simulink model "RealLifeTrainModel"  (R2024a)
settings: Solver=ode1  StartTime=0.0  StopTime=Inf  FixedStep=0.001  RelTol=1e-3
PostLoadFcn:
  | , if any(exist('dsrtsu_mdlpostloadfcn', 'file') ~= 0), dsrtsu_mdlpostloadfcn('Execute', bdroot); end,
InitFcn:
  | , if any(exist('rtifpga_mdlclblib', 'file') ~= 0), rtifpga_mdlclblib('Init', bdroot); end,
undefined symbols (not defined in the file): DiscIntNeverNeededParam
libraries: deeplib x29, svdutilitieslib x28, simulink x8, eeGeneralControl x8, rti1202lib_adc_class1 x6, rti1202serlib x5, spsEdgeDetectorLib x5, rtiemclib x2, rti1202lib_dac_class1 x1
(part 3 of 8)

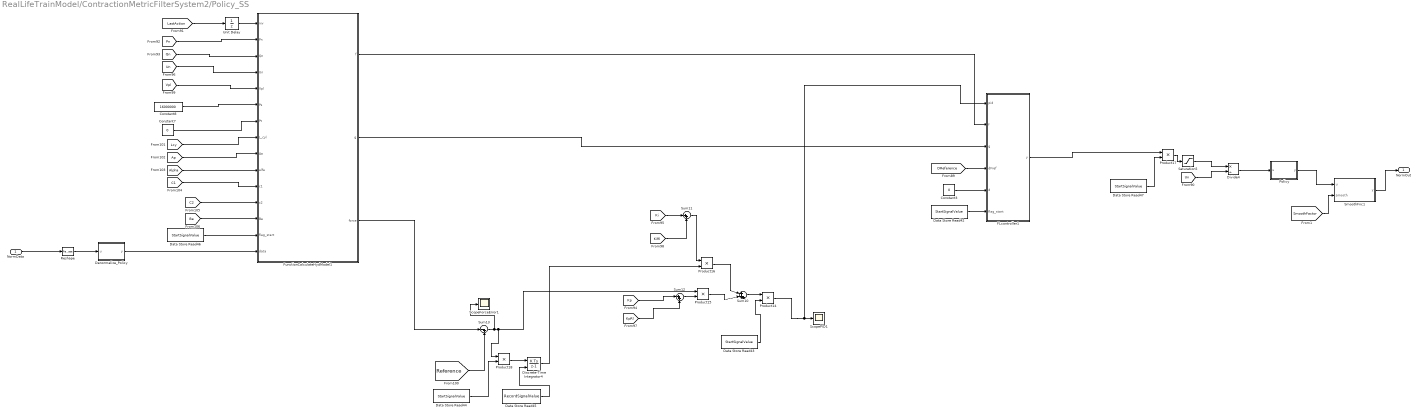
== system RealLifeTrainModel/ContractionMetricFilterSystem2/Policy_SS ==
  NormData : Inport
  Constant3 : Constant  Value=0
  Constant7 : Constant  Value=0
  Constant8 : Constant  Value=16000000
  Data Store Read{42..44,46..47} (5 alike) : DataStoreRead  DataStoreName=StartSignalValue  IndexOptions=Index vector (dialog)  Indices=1  OutputSizes=1
  Data Store Read45 : DataStoreRead  DataStoreName=RecordSignalValue  IndexOptions=Index vector (dialog)  Indices=1  OutputSizes=1
  Denormalize_Policy : MATLAB Function  TreatAsAtomicUnit=on
  Discrete-Time Integrator4 : DiscreteIntegrator  ExternalReset=falling  SampleTime=-1  ICPrevOutput=DiscIntNeverNeededParam  ICPrevScaledInput=DiscIntNeverNeededParam
  Divide4 : Product  Inputs=*/
  FLcontroller1 : MATLAB Function  TreatAsAtomicUnit=on
  FunctionCalculateHydModel1 : MATLAB Function  TreatAsAtomicUnit=on
  Policy : MATLAB Function  TreatAsAtomicUnit=on
  Product{14..18} (5 alike) : Product
  Reshape : Reshape  OutputDimensionality=Row vector (2-D)  OutputDimensions=[8,1]
  Saturation5 : Saturate  UpperLimit=str2num(get_param('Teste_PID/Un','Value'))/str2num(get_param('Teste_PID/SaturationDivider','Value'))  LowerLimit=-str2num(get_param('Teste_PID/Un','Value'))/str2num(get_param('Teste_PID/SaturationDivider','Value'))
  ScopeForceError1 : Scope
  ScopePID1 : Scope
  SmoothFnc1 : MATLAB Function  TreatAsAtomicUnit=on
  Sum10 : Sum  Inputs=|+++
  Sum11 : Sum  Inputs=|++
  Sum12 : Sum  Inputs=|++
  Sum13 : Sum  Inputs=|-+
  Unit Delay : UnitDelay  SampleTime=-1  HasFrameUpgradeWarning=on
  NormOut : Outport
  wires:
  FunctionCalculateHydModel1/3(force) -> Sum13/1
  [Vpl] -> FunctionCalculateHydModel1/5(Vpl)
  Data Store Read45/1 -> Discrete-Time Integrator4/2
  Sum13/1 -> ScopeForceError1/1, Product15/1, Product18/1
  [Alpha] -> FunctionCalculateHydModel1/10(alfa)
  [C2] -> FunctionCalculateHydModel1/12(c2)
  Data Store Read42/1 -> FLcontroller1/6(flag_start)
  [Be] -> FunctionCalculateHydModel1/13(Be)
  [Lcy] -> FunctionCalculateHydModel1/8(L_cyl)
  Data Store Read43/1 -> Product14/2
  [Ap] -> FunctionCalculateHydModel1/9(Aa)
  Product15/1 -> Sum10/2
  Data Store Read44/1 -> Product18/2
  Product18/1 -> Discrete-Time Integrator4/1
  [KpRl] -> Sum12/2
  [Reference] -> Sum13/2
  Constant8/1 -> FunctionCalculateHydModel1/6(Ps)
  Product14/1 -> FLcontroller1/1(pid), ScopePID1/1
  Sum11/1 -> Product16/1
  Sum12/1 -> Product15/2
  Saturation5/1 -> Divide4/1
  [Un] -> Divide4/2
  FLcontroller1/1(y) -> Product17/1
  Denormalize_Policy/1(y) -> FunctionCalculateHydModel1/15(data)
  Sum10/1 -> Product14/1
  [C1] -> FunctionCalculateHydModel1/11(c1)
  Discrete-Time Integrator4/1 -> Product16/2
  [Pn] -> FunctionCalculateHydModel1/2(Pn)
  [LastAction] -> Unit Delay/1
  [Kp] -> Sum12/1
  [Ki] -> Sum11/1
  Constant7/1 -> FunctionCalculateHydModel1/7(Pt)
  Divide4/1 -> Policy/1(u)
  [Qn] -> FunctionCalculateHydModel1/3(Qn)
  Constant3/1 -> FLcontroller1/5(d)
  [KiRl] -> Sum11/2
  Data Store Read47/1 -> Product17/2
  Product16/1 -> Sum10/1
  FunctionCalculateHydModel1/2(g) -> FLcontroller1/3(g)
  Product17/1 -> Saturation5/1
  [DReference] -> FLcontroller1/4(dFref)
  FunctionCalculateHydModel1/1(f) -> FLcontroller1/2(f)
  [Un] -> FunctionCalculateHydModel1/4(Un)
  Data Store Read46/1 -> FunctionCalculateHydModel1/14(flag_start)
  NormData/1 -> Reshape/1
  Reshape/1 -> Denormalize_Policy/1(u)
  Unit Delay/1 -> FunctionCalculateHydModel1/1(ixv)
  [SmoothFactor] -> SmoothFnc1/2(smooth)
  Policy/1(y) -> SmoothFnc1/1(u)
  SmoothFnc1/1(y) -> NormOut/1

== system RealLifeTrainModel/ContractionMetricFilterSystem3/CalcK ==
  State : Inport
  Constant : Constant
  Constant1 : Constant  Value=2
  Constant2 : Constant  Value=3
  Constant3 : Constant  Value=4
  Constant4 : Constant  Value=5
  Constant5 : Constant  Value=6
  Constant6 : Constant  Value=7
  Constant7 : Constant  Value=8
  IndidualGrad1 : Subsystem
  IndidualGrad10 : Subsystem
  IndidualGrad2 : Subsystem
  IndidualGrad3 : Subsystem
  IndidualGrad4 : Subsystem
  IndidualGrad5 : Subsystem
  IndidualGrad6 : Subsystem
  IndidualGrad7 : Subsystem
  Mux : Mux  Inputs=8
  Policy_SS1 : Subsystem
  Reshape8 : Reshape  OutputDimensionality=Customize  OutputDimensions=[1,8]
  K : Outport
  wires:
  State/1 -> Policy_SS1/1(NormData), IndidualGrad7/1(State), IndidualGrad6/1(State), IndidualGrad5/1(State), IndidualGrad4/1(State), IndidualGrad3/1(State), IndidualGrad2/1(State), IndidualGrad1/1(State), IndidualGrad10/1(State)
  Constant/1 -> IndidualGrad10/2(Position)
  Mux/1 -> Reshape8/1
  Constant1/1 -> IndidualGrad1/2(Position)
  Constant2/1 -> IndidualGrad2/2(Position)
  Constant3/1 -> IndidualGrad3/2(Position)
  Constant4/1 -> IndidualGrad4/2(Position)
  Constant5/1 -> IndidualGrad5/2(Position)
  Constant6/1 -> IndidualGrad6/2(Position)
  Constant7/1 -> IndidualGrad7/2(Position)
  Policy_SS1/1(NormOut) -> IndidualGrad6/3(StartValue), IndidualGrad7/3(StartValue), IndidualGrad5/3(StartValue), IndidualGrad4/3(StartValue), IndidualGrad3/3(StartValue), IndidualGrad2/3(StartValue), IndidualGrad1/3(StartValue), IndidualGrad10/3(StartValue)
  IndidualGrad10/1(Grad) -> Mux/1
  IndidualGrad1/1(Grad) -> Mux/2
  IndidualGrad2/1(Grad) -> Mux/3
  IndidualGrad3/1(Grad) -> Mux/4
  IndidualGrad4/1(Grad) -> Mux/5
  IndidualGrad5/1(Grad) -> Mux/6
  IndidualGrad6/1(Grad) -> Mux/7
  IndidualGrad7/1(Grad) -> Mux/8
  Reshape8/1 -> K/1

== system RealLifeTrainModel/ContractionMetricFilterSystem3/Calc_A_B ==
  state : Inport
  Current : Inport  Port=2
  Calc_A_Grad : Subsystem
  A : Outport
  B : Outport  Port=2
  ModelPredict : Outport  Port=3
  wires:
  state/1 -> Calc_A_Grad/1(State)
  Calc_A_Grad/1(A) -> A/1
  Calc_A_Grad/2(B) -> B/1
  Current/1 -> Calc_A_Grad/2(Curent)
  Calc_A_Grad/3(ModelPredict) -> ModelPredict/1

== system RealLifeTrainModel/ContractionMetricFilterSystem3/Mdot_subsystem ==
  StartMetric : Inport
  State : Inport  Port=2
  NextState : Inport  Port=3
  Constant : Constant
  Constant1 : Constant  Value=2
  Constant2 : Constant  Value=3
  Constant3 : Constant  Value=4
  Constant4 : Constant  Value=5
  Constant5 : Constant  Value=6
  Constant6 : Constant  Value=7
  Constant7 : Constant  Value=8
  ConvertMatrix : MATLAB Function  TreatAsAtomicUnit=on
  Demux : Demux  Outputs=8
  Discrete Derivative : simulink/Discrete/Discrete Derivative  gainval=1.0  ICPrevScaledInput=0.0  OutMin=[]  OutMax=[]  OutDataType=fixdt(1, 16)  OutScaling=2^-10  DoSatur=off
  IndidualGrad1 : Subsystem
  IndidualGrad10 : Subsystem
  IndidualGrad2 : Subsystem
  IndidualGrad3 : Subsystem
  IndidualGrad4 : Subsystem
  IndidualGrad5 : Subsystem
  IndidualGrad6 : Subsystem
  IndidualGrad7 : Subsystem
  Product{,1..7} (8 alike) : Product
  Sum : Sum  Inputs=|++++++++
  Mdot : Outport
  wires:
  Constant/1 -> IndidualGrad10/2(Position)
  StartMetric/1 -> ConvertMatrix/1(M_flat)
  State/1 -> Discrete Derivative/1, IndidualGrad7/1(State), IndidualGrad6/1(State), IndidualGrad5/1(State), IndidualGrad4/1(State), IndidualGrad3/1(State), IndidualGrad2/1(State), IndidualGrad1/1(State), IndidualGrad10/1(State)
  Constant1/1 -> IndidualGrad1/2(Position)
  Constant2/1 -> IndidualGrad2/2(Position)
  Constant3/1 -> IndidualGrad3/2(Position)
  Constant4/1 -> IndidualGrad4/2(Position)
  Constant5/1 -> IndidualGrad5/2(Position)
  Constant6/1 -> IndidualGrad6/2(Position)
  Constant7/1 -> IndidualGrad7/2(Position)
  Demux/1 -> [State1]
  Demux/8 -> [State8]
  Demux/7 -> [State7]
  Demux/6 -> [State6]
  Demux/5 -> [State5]
  Demux/4 -> [State4]
  Demux/3 -> [State3]
  Demux/2 -> [State2]
  [State1] -> Product/1
  IndidualGrad10/1(Grad) -> Product/2
  Product/1 -> Sum/1
  [State2] -> Product1/1
  IndidualGrad1/1(Grad) -> Product1/2
  Product1/1 -> Sum/2
  [State3] -> Product2/1
  IndidualGrad2/1(Grad) -> Product2/2
  Product2/1 -> Sum/3
  [State4] -> Product3/1
  IndidualGrad3/1(Grad) -> Product3/2
  Product3/1 -> Sum/4
  [State5] -> Product4/1
  IndidualGrad4/1(Grad) -> Product4/2
  Product4/1 -> Sum/5
  [State6] -> Product5/1
  IndidualGrad5/1(Grad) -> Product5/2
  Product5/1 -> Sum/6
  [State7] -> Product6/1
  [State8] -> Product7/1
  IndidualGrad6/1(Grad) -> Product6/2
  Product6/1 -> Sum/7
  IndidualGrad7/1(Grad) -> Product7/2
  Product7/1 -> Sum/8
  ConvertMatrix/1(M) -> IndidualGrad7/3(StartValue), IndidualGrad6/3(StartValue), IndidualGrad5/3(StartValue), IndidualGrad4/3(StartValue), IndidualGrad3/3(StartValue), IndidualGrad2/3(StartValue), IndidualGrad1/3(StartValue), IndidualGrad10/3(StartValue)
  Sum/1 -> Mdot/1
  NextState/1 -> Demux/1

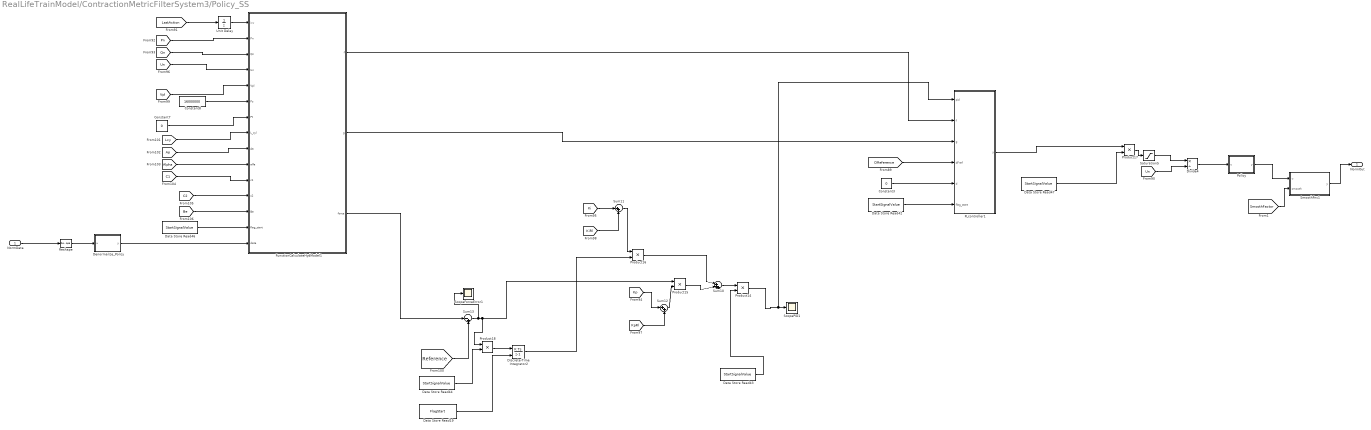
== system RealLifeTrainModel/ContractionMetricFilterSystem3/Policy_SS ==
  NormData : Inport
  Constant3 : Constant  Value=0
  Constant7 : Constant  Value=0
  Constant8 : Constant  Value=16000000
  Data Store Read19 : DataStoreRead  DataStoreName=FlagStart  IndexOptions=Index vector (dialog)  Indices=1  OutputSizes=1
  Data Store Read{42..44,46..47} (5 alike) : DataStoreRead  DataStoreName=StartSignalValue  IndexOptions=Index vector (dialog)  Indices=1  OutputSizes=1
  Denormalize_Policy : MATLAB Function  TreatAsAtomicUnit=on
  Discrete-Time Integrator2 : DiscreteIntegrator  ExternalReset=either  SampleTime=-1  ICPrevOutput=DiscIntNeverNeededParam  ICPrevScaledInput=DiscIntNeverNeededParam
  Divide4 : Product  Inputs=*/
  FLcontroller1 : MATLAB Function  TreatAsAtomicUnit=on
  FunctionCalculateHydModel1 : MATLAB Function  TreatAsAtomicUnit=on
  Policy : MATLAB Function  TreatAsAtomicUnit=on
  Product{14..18} (5 alike) : Product
  Reshape : Reshape  OutputDimensionality=Row vector (2-D)  OutputDimensions=[8,1]
  Saturation5 : Saturate  UpperLimit=str2num(get_param('Teste_PID/Un','Value'))/str2num(get_param('Teste_PID/SaturationDivider','Value'))  LowerLimit=-str2num(get_param('Teste_PID/Un','Value'))/str2num(get_param('Teste_PID/SaturationDivider','Value'))
  ScopeForceError1 : Scope
  ScopePID1 : Scope
  SmoothFnc1 : MATLAB Function  TreatAsAtomicUnit=on
  Sum10 : Sum  Inputs=|+++
  Sum11 : Sum  Inputs=|++
  Sum12 : Sum  Inputs=|++
  Sum13 : Sum  Inputs=|-+
  Unit Delay : UnitDelay  SampleTime=-1  HasFrameUpgradeWarning=on
  NormOut : Outport
  wires:
  FunctionCalculateHydModel1/3(force) -> Sum13/1
  [Vpl] -> FunctionCalculateHydModel1/5(Vpl)
  Sum13/1 -> ScopeForceError1/1, Product15/1, Product18/1
  [Alpha] -> FunctionCalculateHydModel1/10(alfa)
  [C2] -> FunctionCalculateHydModel1/12(c2)
  Data Store Read42/1 -> FLcontroller1/6(flag_start)
  [Be] -> FunctionCalculateHydModel1/13(Be)
  [Lcy] -> FunctionCalculateHydModel1/8(L_cyl)
  Data Store Read43/1 -> Product14/2
  [Ap] -> FunctionCalculateHydModel1/9(Aa)
  Product15/1 -> Sum10/2
  Data Store Read44/1 -> Product18/2
  Product18/1 -> Discrete-Time Integrator2/1
  [KpRl] -> Sum12/2
  [Reference] -> Sum13/2
  Constant8/1 -> FunctionCalculateHydModel1/6(Ps)
  Product14/1 -> FLcontroller1/1(pid), ScopePID1/1
  Sum11/1 -> Product16/1
  Sum12/1 -> Product15/2
  Saturation5/1 -> Divide4/1
  [Un] -> Divide4/2
  FLcontroller1/1(y) -> Product17/1
  Denormalize_Policy/1(y) -> FunctionCalculateHydModel1/15(data)
  Sum10/1 -> Product14/1
  [C1] -> FunctionCalculateHydModel1/11(c1)
  Discrete-Time Integrator2/1 -> Product16/2
  [Pn] -> FunctionCalculateHydModel1/2(Pn)
  [LastAction] -> Unit Delay/1
  [Kp] -> Sum12/1
  [Ki] -> Sum11/1
  Constant7/1 -> FunctionCalculateHydModel1/7(Pt)
  Divide4/1 -> Policy/1(u)
  [Qn] -> FunctionCalculateHydModel1/3(Qn)
  Constant3/1 -> FLcontroller1/5(d)
  [KiRl] -> Sum11/2
  Data Store Read47/1 -> Product17/2
  Product16/1 -> Sum10/1
  FunctionCalculateHydModel1/2(g) -> FLcontroller1/3(g)
  Product17/1 -> Saturation5/1
  [DReference] -> FLcontroller1/4(dFref)
  FunctionCalculateHydModel1/1(f) -> FLcontroller1/2(f)
  [Un] -> FunctionCalculateHydModel1/4(Un)
  Data Store Read46/1 -> FunctionCalculateHydModel1/14(flag_start)
  NormData/1 -> Reshape/1
  Reshape/1 -> Denormalize_Policy/1(u)
  Unit Delay/1 -> FunctionCalculateHydModel1/1(ixv)
  [SmoothFactor] -> SmoothFnc1/2(smooth)
  Policy/1(y) -> SmoothFnc1/1(u)
  SmoothFnc1/1(y) -> NormOut/1
  Data Store Read19/1 -> Discrete-Time Integrator2/2

== system RealLifeTrainModel/RTI Data/RTI Data Store ==
  RTI Data Store : Subsystem  mask(RTI_DATA_STORE){}
      mask help:
      | RTI Data Store Block. This block is used by RTI to store internal model dependent data. Deleting this block will result in data loss.
      |
      | NEVER DELETE, COPY, OR MODIFY THIS BLOCK!
      mask Help:
      | RTI Data Store Block. This block is used by RTI to store internal model dependent data. Deleting this block will result in data loss.
      | 
      | NEVER DELETE, COPY, OR MODIFY THIS BLOCK!
      mask Display: text(0.5, 0.5, ' ', 'HorizontalAlignment', 'center');

== system RealLifeTrainModel/CommSystem/SendMessageSystem/CancelSubsystem ==
  CancelCounter : Inport
  CancelLimit : Inport  Port=2
  Action Port : ActionPort  ActionPortLabel="if(u1  == 1)"
  Data Store Write1 : DataStoreWrite  DataStoreName=CancelCounter  IndexOptions=Index vector (dialog)  Indices=1  OutputSizes=1
  If : If
  If Action Subsystem : Subsystem  TreatAsAtomicUnit=on
  MATLAB Function : MATLAB Function  TreatAsAtomicUnit=on
  ScopeCancelCounter : Scope
  wires:
  CancelCounter/1 -> ScopeCancelCounter/1, MATLAB Function/1(counter)
  CancelLimit/1 -> MATLAB Function/2(limit)
  MATLAB Function/2(new_counter) -> Data Store Write1/1
  MATLAB Function/1(cancel) -> If/1
  If/1 -> If Action Subsystem/Action

== system RealLifeTrainModel/CommSystem/SendMessageSystem/If Action Subsystem ==
  Action Port : ActionPort  ActionPortLabel=else
  Constant : Constant
  Constant1 : Constant  Value=0
  Constant3 : Constant  Value=0
  Data Store Write : DataStoreWrite  DataStoreName=CancelCounter  IndexOptions=Index vector (dialog)  Indices=1  OutputSizes=1
  Data Store Write2 : DataStoreWrite  DataStoreName=Counter  IndexOptions=Index vector (dialog)  Indices=1  OutputSizes=1
  Out1 : Outport
  wires:
  Constant/1 -> Out1/1
  Constant3/1 -> Data Store Write2/1
  Constant1/1 -> Data Store Write/1

== system RealLifeTrainModel/CommSystem/SendMessageSystem/If Action Subsystem1 ==
  Action Port : ActionPort  ActionPortLabel=else

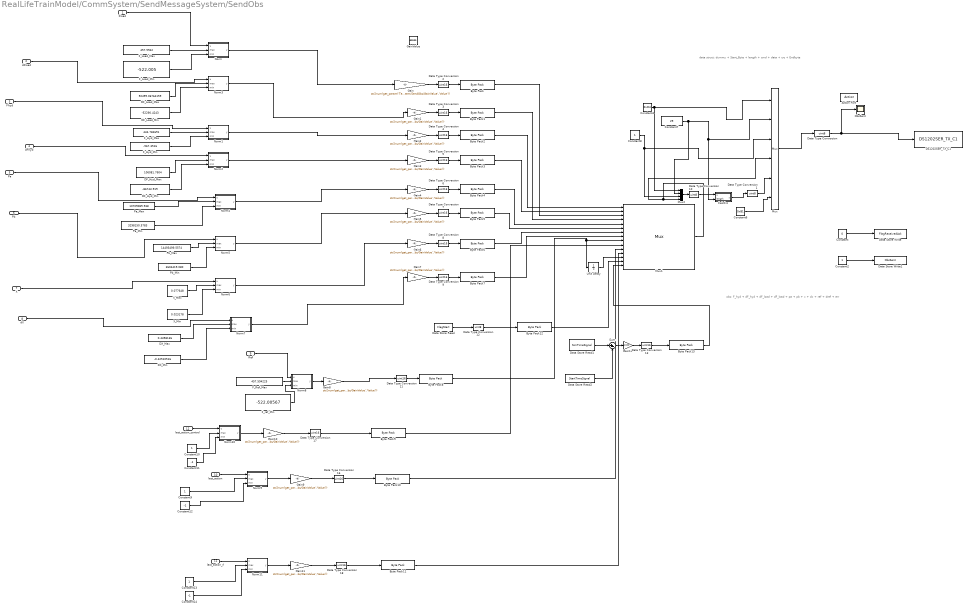
== system RealLifeTrainModel/CommSystem/SendMessageSystem/SendObs ==
  note: data struct: dummy + Start_Byte + length + cmd + data + crc + Endbyte
  note: obs: F_hyd + dF_hyd + dF_load + dF_load + pa + pb + x + dx + ref + dref + err
  Fload : Inport
  dFload : Inport  Port=2
  Fhyd : Inport  Port=3
  dFhyd : Inport  Port=4
  Pa : Inport  Port=5
  Pb : Inport  Port=6
  X : Inport  Port=7
  dX : Inport  Port=8
  Ref : Inport  Port=9
  last_action : Inport  Port=10
  last_action_rl : Inport  Port=11
  last_action_control : Inport  Port=12
  Action Port : ActionPort  ActionPortLabel="if(u1  == 1)"
  Byte Pack{,1..11,13} (13 alike) : svdutilitieslib/Byte Pack  maskPackedDataType=uint8  datatypes={'uint16'}  byteAlign=1  blockPlatform=tic2000
  Byte Pack12 : svdutilitieslib/Byte Pack  maskPackedDataType=uint8  datatypes={'uint8'}  byteAlign=1  blockPlatform=tic2000
  CalcCrc : MATLAB Function  TreatAsAtomicUnit=on
  Constant : Constant  Value=0  OutDataTypeStr=uint8
  Constant10 : Constant
  Constant11 : Constant  Value=-1
  Constant12 : Constant  Value=-1
  Constant13 : Constant
  Constant14 : Constant  Value=-1
  Constant2 : Constant  OutDataTypeStr=uint8
  Constant4 : Constant  Value=0xD4  OutDataTypeStr=uint8
  Constant6 : Constant  Value=0xB1  OutDataTypeStr=uint8
  Constant7 : Constant  Value=29  OutDataTypeStr=uint8
  Constant8 : Constant  OutDataTypeStr=uint8
  Constant9 : Constant
  DF_Hyd_Max : Constant  Value=106081.7604
  DF_Hyd_Min : Constant  Value=-86743.919
  DF_Load_Max : Constant  Value=50499.06764159
  DF_Load_Min : Constant  Value=-52290.4243
  DS1202SER_TX_C1 : rti1202serlib/DS1202SER_TX_C1  Reserved1=[]  Reserved2=[]  Reserved3=[]  Reserved4=[]  DSProperties=struct('RTI',struct('IOBoardType',{{'DS1202','SER'}},'SlaveProcessor','NONE','Version',uint32(1),'BlockType',struct('isSLSource',uint8(1),'isSLSink',uint8(1),'isHWSource',uint8(1),'isHWSink',uint8(0),'isSetup',uint8(0),'isInline',uint8(1),'isNonInline',uint8(0),'isInterrupt',uint8(0),'isChannelwise',uint8(1)),'UnitType','GENSER','Identifier','TRANSMIT','DialogType','ML','BlockSet','NONE'))  RTIBlockInterface=struct('BlockName',struct('Token',{{'DS1202SER_TX_C'}},'BlockParam',{{'ChannelNo'}}),'InputPortsWidth',int32([34 1]),'InputPortsActive',[1 0],'InputPortsDataType',{{'SS_UINT8','SS_UINT32'}},'InputPortsName',{{'TXBytes','NumBytes'}},'OutputPortsWidth',int32([1 1]),'OutputPortsActive',[0 0],'OutputPortsDataType',{{'SS_UINT32','SS_INT32'}},'OutputPortsName',{{'NumTXBytes','Status'}},'BlockDisplay',{{['Serial Transmit'],'center'}},'IconTransparency','on','ParameterTunableNames',{{}},'InitLevel',2,'DialogFcn','guigensertransmit','MaskDescription',['To write data to the UART SW FIFO.'])  RTIBlockParameters=struct('BoardNo',{{1,'ON',[1 1]}},'ChannelNo',{{1,'ON',[1 2]}},'ChannelNumOf',{{2,'OFF',[]}},'TransmitFifoOverrunMode',{{1,'OFF',[]}},'ParamTunableMode',{{2,'OFF',[]}},'BytesRefNumOfT',{{'1','OFF',[1 inf]}},'BytesRefNumOfNT',{{'34','OFF',[1 inf]}},'BytesRefNumOfMax',{{'15','OFF',[1 inf]}},'BytesRefNumOfMode',{{0,'OFF',[]}},'BytesActNumOfMode',{{0,'OFF',[]}},'TransmissionStatusMode',{{0,'OFF',[]}},'FifoSizeDefault',{{64,'OFF',[]}},'TLCFileName',{{'rtigensertransmit','OFF',[]}})  RTISFcnParameters=struct('BoardNo','double','ChannelNo','double','ChannelNumOf','double','TransmitFifoOverrunMode','double','ParamTunableMode','double','BytesRefNumOfT','double','BytesRefNumOfNT','double','BytesRefNumOfMax','double','BytesRefNumOfMode','double','BytesActNumOfMode','double','TransmissionStatusMode','double','TLCFileName','char')  RTIBlockParaDefault=struct('BoardNo',1,'ChannelNo',1,'ChannelNumOf',2,'TransmitFifoOverrunMode',1,'ParamTunableMode',1,'BytesRefNumOfT',1,'BytesRefNumOfNT',1,'BytesRefNumOfMax',1,'BytesRefNumOfMode',0,'BytesActNumOfMode',1,'TransmissionStatusMode',1,'FifoSizeDefault',64,'TLCFileName','rtigensertransmit')
  DX_Max : Constant  Value=0.4358136
  DX_Min : Constant  Value=-0.42510516
  Data Store Read : DataStoreRead  DataStoreName=FlagStart  IndexOptions=Index vector (dialog)  Indices=1  OutputSizes=1
  Data Store Read1 : DataStoreRead  DataStoreName=SimTimeSignal  IndexOptions=Index vector (dialog)  Indices=1  OutputSizes=1
  Data Store Read2 : DataStoreRead  DataStoreName=StartTimeSignal  IndexOptions=Index vector (dialog)  Indices=1  OutputSizes=1
  Data Store Write : DataStoreWrite  DataStoreName=FlagReceivedAck  IndexOptions=Index vector (dialog)  Indices=1  OutputSizes=1
  Data Store Write1 : DataStoreWrite  DataStoreName=ObsSent  IndexOptions=Index vector (dialog)  Indices=1  OutputSizes=1
  Data Type Conversion{,1,10,12} (4 alike) : DataTypeConversion  OutDataTypeStr=uint8
  Data Type Conversion{2..9,11,13,16..18} (13 alike) : DataTypeConversion  OutDataTypeStr=uint16
  F_Hyd_Max : Constant  Value=434.784691
  F_Hyd_Min : Constant  Value=-567.3516
  F_Load_Max : Constant  Value=457.5942
  F_Load_Min : Constant  Value=-522.005
  F_Ref_Max : Constant  Value=457.594225
  F_ref_Min : Constant  Value=-522.00567
  Gain{,1..11} (12 alike) : Gain  Gain=str2num(get_param('Teste_PID/CommSystem/SendMessageSystem/SendObs/GainValue','Value'))
  Gain12 : Gain  Gain=1000
  GainValue : Constant  Value=65535
  Mux : Mux  Inputs=6
  Mux1 : Mux  Inputs=15
  Mux2 : Mux
  Norm : MATLAB Function  TreatAsAtomicUnit=on
  Norm1 : MATLAB Function  TreatAsAtomicUnit=on
  Norm10 : MATLAB Function  TreatAsAtomicUnit=on
  Norm11 : MATLAB Function  TreatAsAtomicUnit=on
  Norm2 : MATLAB Function  TreatAsAtomicUnit=on
  Norm3 : MATLAB Function  TreatAsAtomicUnit=on
  Norm4 : MATLAB Function  TreatAsAtomicUnit=on
  Norm5 : MATLAB Function  TreatAsAtomicUnit=on
  Norm6 : MATLAB Function  TreatAsAtomicUnit=on
  Norm7 : MATLAB Function  TreatAsAtomicUnit=on
  Norm8 : MATLAB Function  TreatAsAtomicUnit=on
  Norm9 : MATLAB Function  TreatAsAtomicUnit=on
  ObsSent : Scope
  Pa_Max : Constant  Value=10709089.938
  Pa_Min : Constant  Value=3298150.5783
  Pb_Max : Constant  Value=14493499.5574
  Pb_Min : Constant  Value=3604419.080
  Sum : Sum  Inputs=|+-
  Unit Delay : UnitDelay  SampleTime=-1  HasFrameUpgradeWarning=on
  X_Max : Constant  Value=0.077648
  X_Min : Constant  Value=0.023178
  wires:
  Constant/1 -> Data Store Write/1
  Constant2/1 -> Data Store Write1/1
  Mux/1 -> Data Type Conversion/1
  Constant7/1 -> Mux2/2, CalcCrc/2(length), Mux/2
  CalcCrc/1(y) -> Data Type Conversion1/1
  Gain/1 -> Data Type Conversion2/1
  Data Type Conversion2/1 -> Byte Pack/1
  Data Type Conversion3/1 -> Byte Pack1/1
  Gain1/1 -> Data Type Conversion3/1
  Gain2/1 -> Data Type Conversion4/1
  Data Type Conversion4/1 -> Byte Pack2/1
  Gain3/1 -> Data Type Conversion5/1
  Data Type Conversion5/1 -> Byte Pack3/1
  Gain4/1 -> Data Type Conversion6/1
  Data Type Conversion6/1 -> Byte Pack4/1
  Gain5/1 -> Data Type Conversion7/1
  Data Type Conversion7/1 -> Byte Pack5/1
  Gain6/1 -> Data Type Conversion8/1
  Data Type Conversion8/1 -> Byte Pack6/1
  Byte Pack6/1 -> Mux1/7
  Byte Pack5/1 -> Mux1/6
  Byte Pack4/1 -> Mux1/5
  Constant4/1 -> Mux2/1, Mux/1
  Mux1/1 -> Mux/4, Mux2/4
  Mux2/1 -> Data Type Conversion10/1
  Data Type Conversion1/1 -> Mux/5
  Constant6/1 -> Mux/6
  Data Type Conversion10/1 -> CalcCrc/1(u)
  Constant8/1 -> Mux/3, Mux2/3
  F_Load_Max/1 -> Norm/2(max)
  F_Load_Min/1 -> Norm/3(min)
  F_Hyd_Max/1 -> Norm1/2(max)
  F_Hyd_Min/1 -> Norm1/3(min)
  DF_Load_Max/1 -> Norm3/2(max)
  DF_Load_Min/1 -> Norm3/3(min)
  DF_Hyd_Max/1 -> Norm2/2(max)
  DF_Hyd_Min/1 -> Norm2/3(min)
  Byte Pack7/1 -> Mux1/8
  Gain7/1 -> Data Type Conversion9/1
  Data Type Conversion9/1 -> Byte Pack7/1
  Pa_Min/1 -> Norm4/3(min)
  Pa_Max/1 -> Norm4/2(max)
  Pb_Min/1 -> Norm5/3(min)
  Pb_Max/1 -> Norm5/2(max)
  X_Max/1 -> Norm6/2(max)
  X_Min/1 -> Norm6/3(min)
  DX_Max/1 -> Norm7/2(max)
  DX_Min/1 -> Norm7/3(min)
  F_Ref_Max/1 -> Norm8/2(max)
  F_ref_Min/1 -> Norm8/3(min)
  Norm8/1(y) -> Gain8/1
  Fload/1 -> Norm/1(u)
  dFload/1 -> Norm3/1(u)
  Fhyd/1 -> Norm1/1(u)
  dFhyd/1 -> Norm2/1(u)
  Pa/1 -> Norm4/1(u)
  Pb/1 -> Norm5/1(u)
  X/1 -> Norm6/1(u)
  dX/1 -> Norm7/1(u)
  Norm/1(y) -> Gain/1
  Norm3/1(y) -> Gain1/1
  Norm1/1(y) -> Gain2/1
  Norm2/1(y) -> Gain3/1
  Norm4/1(y) -> Gain4/1
  Norm5/1(y) -> Gain5/1
  Norm6/1(y) -> Gain6/1
  Norm7/1(y) -> Gain7/1
  Gain8/1 -> Data Type Conversion11/1
  Data Type Conversion11/1 -> Byte Pack8/1
  Byte Pack8/1 -> Unit Delay/1, Mux1/9
  Ref/1 -> Norm8/1(u)
  Byte Pack2/1 -> Mux1/1
  Byte Pack3/1 -> Mux1/2
  Byte Pack/1 -> Mux1/3
  Byte Pack1/1 -> Mux1/4
  last_action/1 -> Norm9/1(u)
  last_action_control/1 -> Norm10/1(u)
  Constant9/1 -> Norm9/2(max)
  Constant10/1 -> Norm10/2(max)
  Constant11/1 -> Norm10/3(min)
  Constant12/1 -> Norm9/3(min)
  Norm9/1(y) -> Gain9/1
  Norm10/1(y) -> Gain10/1
  last_action_rl/1 -> Norm11/1(u)
  Constant13/1 -> Norm11/2(max)
  Constant14/1 -> Norm11/3(min)
  Norm11/1(y) -> Gain11/1
  Gain9/1 -> Data Type Conversion16/1
  Gain10/1 -> Data Type Conversion17/1
  Gain11/1 -> Data Type Conversion18/1
  Data Type Conversion17/1 -> Byte Pack9/1
  Data Type Conversion16/1 -> Byte Pack10/1
  Data Type Conversion18/1 -> Byte Pack11/1
  Data Type Conversion/1 -> DS1202SER_TX_C1/1, ObsSent/1
  Byte Pack9/1 -> Mux1/10
  Byte Pack10/1 -> Mux1/11
  Byte Pack11/1 -> Mux1/12
  Unit Delay/1 -> Mux1/13
  Data Store Read/1 -> Data Type Conversion12/1
  Data Type Conversion12/1 -> Byte Pack12/1
  Byte Pack12/1 -> Mux1/14
  Data Store Read1/1 -> Sum/1
  Data Store Read2/1 -> Sum/2
  Sum/1 -> Gain12/1
  Gain12/1 -> Data Type Conversion13/1
  Data Type Conversion13/1 -> Byte Pack13/1
  Byte Pack13/1 -> Mux1/15

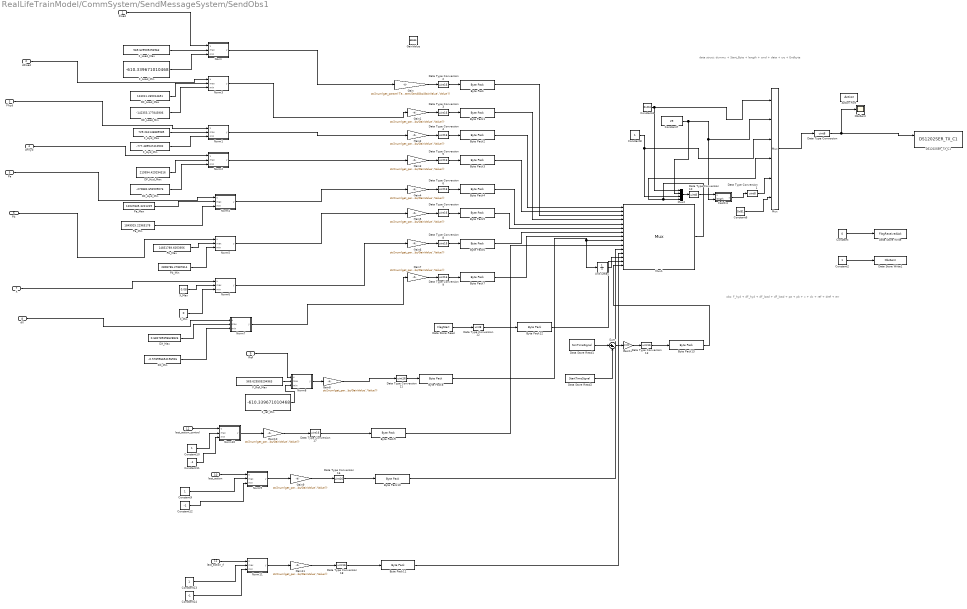
== system RealLifeTrainModel/CommSystem/SendMessageSystem/SendObs1 ==
  note: data struct: dummy + Start_Byte + length + cmd + data + crc + Endbyte
  note: obs: F_hyd + dF_hyd + dF_load + dF_load + pa + pb + x + dx + ref + dref + err
  Fload : Inport
  dFload : Inport  Port=2
  Fhyd : Inport  Port=3
  dFhyd : Inport  Port=4
  Pa : Inport  Port=5
  Pb : Inport  Port=6
  X : Inport  Port=7
  dX : Inport  Port=8
  Ref : Inport  Port=9
  last_action : Inport  Port=10
  last_action_rl : Inport  Port=11
  last_action_control : Inport  Port=12
  Action Port : ActionPort
  Byte Pack{,1..11,13} (13 alike) : svdutilitieslib/Byte Pack  maskPackedDataType=uint8  datatypes={'uint16'}  byteAlign=1  blockPlatform=tic2000
  Byte Pack12 : svdutilitieslib/Byte Pack  maskPackedDataType=uint8  datatypes={'uint8'}  byteAlign=1  blockPlatform=tic2000
  CalcCrc : MATLAB Function  TreatAsAtomicUnit=on
  Constant : Constant  Value=0  OutDataTypeStr=uint8
  Constant10 : Constant
  Constant11 : Constant  Value=-1
  Constant12 : Constant  Value=-1
  Constant13 : Constant
  Constant14 : Constant  Value=-1
  Constant2 : Constant  OutDataTypeStr=uint8
  Constant4 : Constant  Value=0xD4  OutDataTypeStr=uint8
  Constant6 : Constant  Value=0xB1  OutDataTypeStr=uint8
  Constant7 : Constant  Value=29  OutDataTypeStr=uint8
  Constant8 : Constant  OutDataTypeStr=uint8
  Constant9 : Constant
  DF_Hyd_Max : Constant  Value=219994.429294316
  DF_Hyd_Min : Constant  Value=-270882.694509076
  DF_Load_Max : Constant  Value=123011.265014651
  DF_Load_Min : Constant  Value=-142353.177843906
  DS1202SER_TX_C1 : rti1202serlib/DS1202SER_TX_C1  Reserved1=[]  Reserved2=[]  Reserved3=[]  Reserved4=[]  DSProperties=struct('RTI',struct('IOBoardType',{{'DS1202','SER'}},'SlaveProcessor','NONE','Version',uint32(1),'BlockType',struct('isSLSource',uint8(1),'isSLSink',uint8(1),'isHWSource',uint8(1),'isHWSink',uint8(0),'isSetup',uint8(0),'isInline',uint8(1),'isNonInline',uint8(0),'isInterrupt',uint8(0),'isChannelwise',uint8(1)),'UnitType','GENSER','Identifier','TRANSMIT','DialogType','ML','BlockSet','NONE'))  RTIBlockInterface=struct('BlockName',struct('Token',{{'DS1202SER_TX_C'}},'BlockParam',{{'ChannelNo'}}),'InputPortsWidth',int32([34 1]),'InputPortsActive',[1 0],'InputPortsDataType',{{'SS_UINT8','SS_UINT32'}},'InputPortsName',{{'TXBytes','NumBytes'}},'OutputPortsWidth',int32([1 1]),'OutputPortsActive',[0 0],'OutputPortsDataType',{{'SS_UINT32','SS_INT32'}},'OutputPortsName',{{'NumTXBytes','Status'}},'BlockDisplay',{{['Serial Transmit'],'center'}},'IconTransparency','on','ParameterTunableNames',{{}},'InitLevel',2,'DialogFcn','guigensertransmit','MaskDescription',['To write data to the UART SW FIFO.'])  RTIBlockParameters=struct('BoardNo',{{1,'ON',[1 1]}},'ChannelNo',{{1,'ON',[1 2]}},'ChannelNumOf',{{2,'OFF',[]}},'TransmitFifoOverrunMode',{{1,'OFF',[]}},'ParamTunableMode',{{2,'OFF',[]}},'BytesRefNumOfT',{{'1','OFF',[1 inf]}},'BytesRefNumOfNT',{{'34','OFF',[1 inf]}},'BytesRefNumOfMax',{{'15','OFF',[1 inf]}},'BytesRefNumOfMode',{{0,'OFF',[]}},'BytesActNumOfMode',{{0,'OFF',[]}},'TransmissionStatusMode',{{0,'OFF',[]}},'FifoSizeDefault',{{64,'OFF',[]}},'TLCFileName',{{'rtigensertransmit','OFF',[]}})  RTISFcnParameters=struct('BoardNo','double','ChannelNo','double','ChannelNumOf','double','TransmitFifoOverrunMode','double','ParamTunableMode','double','BytesRefNumOfT','double','BytesRefNumOfNT','double','BytesRefNumOfMax','double','BytesRefNumOfMode','double','BytesActNumOfMode','double','TransmissionStatusMode','double','TLCFileName','char')  RTIBlockParaDefault=struct('BoardNo',1,'ChannelNo',1,'ChannelNumOf',2,'TransmitFifoOverrunMode',1,'ParamTunableMode',1,'BytesRefNumOfT',1,'BytesRefNumOfNT',1,'BytesRefNumOfMax',1,'BytesRefNumOfMode',0,'BytesActNumOfMode',1,'TransmissionStatusMode',1,'FifoSizeDefault',64,'TLCFileName','rtigensertransmit')
  DX_Max : Constant  Value=0.682789396628826
  DX_Min : Constant  Value=-0.578996654196926
  Data Store Read : DataStoreRead  DataStoreName=FlagStart  IndexOptions=Index vector (dialog)  Indices=1  OutputSizes=1
  Data Store Read1 : DataStoreRead  DataStoreName=SimTimeSignal  IndexOptions=Index vector (dialog)  Indices=1  OutputSizes=1
  Data Store Read2 : DataStoreRead  DataStoreName=StartTimeSignal  IndexOptions=Index vector (dialog)  Indices=1  OutputSizes=1
  Data Store Write : DataStoreWrite  DataStoreName=FlagReceivedAck  IndexOptions=Index vector (dialog)  Indices=1  OutputSizes=1
  Data Store Write1 : DataStoreWrite  DataStoreName=ObsSent  IndexOptions=Index vector (dialog)  Indices=1  OutputSizes=1
  Data Type Conversion{,1,10,12} (4 alike) : DataTypeConversion  OutDataTypeStr=uint8
  Data Type Conversion{2..9,11,13,16..18} (13 alike) : DataTypeConversion  OutDataTypeStr=uint16
  F_Hyd_Max : Constant  Value=729.261146885585
  F_Hyd_Min : Constant  Value=-777.489547410502
  F_Load_Max : Constant  Value=569.629505294963
  F_Load_Min : Constant  Value=-610.339671010468
  F_Ref_Max : Constant  Value=569.629505294963
  F_ref_Min : Constant  Value=-610.339671010468
  Gain{,1..11} (12 alike) : Gain  Gain=str2num(get_param('Teste_PID/CommSystem/SendMessageSystem/SendObs/GainValue','Value'))
  Gain12 : Gain  Gain=1000
  GainValue : Constant  Value=65535
  Mux : Mux  Inputs=6
  Mux1 : Mux  Inputs=15
  Mux2 : Mux
  Norm : MATLAB Function  TreatAsAtomicUnit=on
  Norm1 : MATLAB Function  TreatAsAtomicUnit=on
  Norm10 : MATLAB Function  TreatAsAtomicUnit=on
  Norm11 : MATLAB Function  TreatAsAtomicUnit=on
  Norm2 : MATLAB Function  TreatAsAtomicUnit=on
  Norm3 : MATLAB Function  TreatAsAtomicUnit=on
  Norm4 : MATLAB Function  TreatAsAtomicUnit=on
  Norm5 : MATLAB Function  TreatAsAtomicUnit=on
  Norm6 : MATLAB Function  TreatAsAtomicUnit=on
  Norm7 : MATLAB Function  TreatAsAtomicUnit=on
  Norm8 : MATLAB Function  TreatAsAtomicUnit=on
  Norm9 : MATLAB Function  TreatAsAtomicUnit=on
  ObsSent : Scope
  Pa_Max : Constant  Value=12037835.3221229
  Pa_Min : Constant  Value=1849925.22965178
  Pb_Max : Constant  Value=14831789.6053956
  Pb_Min : Constant  Value=2808786.27887814
  Sum : Sum  Inputs=|+-
  Unit Delay : UnitDelay  SampleTime=-1  HasFrameUpgradeWarning=on
  X_Max : Constant  Value=0.08
  X_Min : Constant  Value=0
  wires:
  Constant/1 -> Data Store Write/1
  Constant2/1 -> Data Store Write1/1
  Mux/1 -> Data Type Conversion/1
  Constant7/1 -> Mux2/2, CalcCrc/2(length), Mux/2
  CalcCrc/1(y) -> Data Type Conversion1/1
  Gain/1 -> Data Type Conversion2/1
  Data Type Conversion2/1 -> Byte Pack/1
  Data Type Conversion3/1 -> Byte Pack1/1
  Gain1/1 -> Data Type Conversion3/1
  Gain2/1 -> Data Type Conversion4/1
  Data Type Conversion4/1 -> Byte Pack2/1
  Gain3/1 -> Data Type Conversion5/1
  Data Type Conversion5/1 -> Byte Pack3/1
  Gain4/1 -> Data Type Conversion6/1
  Data Type Conversion6/1 -> Byte Pack4/1
  Gain5/1 -> Data Type Conversion7/1
  Data Type Conversion7/1 -> Byte Pack5/1
  Gain6/1 -> Data Type Conversion8/1
  Data Type Conversion8/1 -> Byte Pack6/1
  Byte Pack6/1 -> Mux1/7
  Byte Pack5/1 -> Mux1/6
  Byte Pack4/1 -> Mux1/5
  Constant4/1 -> Mux2/1, Mux/1
  Mux1/1 -> Mux/4, Mux2/4
  Mux2/1 -> Data Type Conversion10/1
  Data Type Conversion1/1 -> Mux/5
  Constant6/1 -> Mux/6
  Data Type Conversion10/1 -> CalcCrc/1(u)
  Constant8/1 -> Mux/3, Mux2/3
  F_Load_Max/1 -> Norm/2(max)
  F_Load_Min/1 -> Norm/3(min)
  F_Hyd_Max/1 -> Norm1/2(max)
  F_Hyd_Min/1 -> Norm1/3(min)
  DF_Load_Max/1 -> Norm3/2(max)
  DF_Load_Min/1 -> Norm3/3(min)
  DF_Hyd_Max/1 -> Norm2/2(max)
  DF_Hyd_Min/1 -> Norm2/3(min)
  Byte Pack7/1 -> Mux1/8
  Gain7/1 -> Data Type Conversion9/1
  Data Type Conversion9/1 -> Byte Pack7/1
  Pa_Min/1 -> Norm4/3(min)
  Pa_Max/1 -> Norm4/2(max)
  Pb_Min/1 -> Norm5/3(min)
  Pb_Max/1 -> Norm5/2(max)
  X_Max/1 -> Norm6/2(max)
  X_Min/1 -> Norm6/3(min)
  DX_Max/1 -> Norm7/2(max)
  DX_Min/1 -> Norm7/3(min)
  F_Ref_Max/1 -> Norm8/2(max)
  F_ref_Min/1 -> Norm8/3(min)
  Norm8/1(y) -> Gain8/1
  Fload/1 -> Norm/1(u)
  dFload/1 -> Norm3/1(u)
  Fhyd/1 -> Norm1/1(u)
  dFhyd/1 -> Norm2/1(u)
  Pa/1 -> Norm4/1(u)
  Pb/1 -> Norm5/1(u)
  X/1 -> Norm6/1(u)
  dX/1 -> Norm7/1(u)
  Norm/1(y) -> Gain/1
  Norm3/1(y) -> Gain1/1
  Norm1/1(y) -> Gain2/1
  Norm2/1(y) -> Gain3/1
  Norm4/1(y) -> Gain4/1
  Norm5/1(y) -> Gain5/1
  Norm6/1(y) -> Gain6/1
  Norm7/1(y) -> Gain7/1
  Gain8/1 -> Data Type Conversion11/1
  Data Type Conversion11/1 -> Byte Pack8/1
  Byte Pack8/1 -> Unit Delay/1, Mux1/9
  Ref/1 -> Norm8/1(u)
  Byte Pack2/1 -> Mux1/1
  Byte Pack3/1 -> Mux1/2
  Byte Pack/1 -> Mux1/3
  Byte Pack1/1 -> Mux1/4
  last_action/1 -> Norm9/1(u)
  last_action_control/1 -> Norm10/1(u)
  Constant9/1 -> Norm9/2(max)
  Constant10/1 -> Norm10/2(max)
  Constant11/1 -> Norm10/3(min)
  Constant12/1 -> Norm9/3(min)
  Norm9/1(y) -> Gain9/1
  Norm10/1(y) -> Gain10/1
  last_action_rl/1 -> Norm11/1(u)
  Constant13/1 -> Norm11/2(max)
  Constant14/1 -> Norm11/3(min)
  Norm11/1(y) -> Gain11/1
  Gain9/1 -> Data Type Conversion16/1
  Gain10/1 -> Data Type Conversion17/1
  Gain11/1 -> Data Type Conversion18/1
  Data Type Conversion17/1 -> Byte Pack9/1
  Data Type Conversion16/1 -> Byte Pack10/1
  Data Type Conversion18/1 -> Byte Pack11/1
  Data Type Conversion/1 -> DS1202SER_TX_C1/1, ObsSent/1
  Byte Pack9/1 -> Mux1/10
  Byte Pack10/1 -> Mux1/11
  Byte Pack11/1 -> Mux1/12
  Unit Delay/1 -> Mux1/13
  Data Store Read/1 -> Data Type Conversion12/1
  Data Type Conversion12/1 -> Byte Pack12/1
  Byte Pack12/1 -> Mux1/14
  Data Store Read1/1 -> Sum/1
  Data Store Read2/1 -> Sum/2
  Sum/1 -> Gain12/1
  Gain12/1 -> Data Type Conversion13/1
  Data Type Conversion13/1 -> Byte Pack13/1
  Byte Pack13/1 -> Mux1/15

== system RealLifeTrainModel/ContractionMetricFilterSystem3/CalcK/IndidualGrad1 ==
  State : Inport
  Position : Inport  Port=2
  StartValue : Inport  Port=3
  MATLAB Function2 : MATLAB Function  TreatAsAtomicUnit=on
  MATLAB Function5 : MATLAB Function  TreatAsAtomicUnit=on
  Policy_SS1 : Subsystem
  Sum4 : Sum  Inputs=|++
  Grad : Outport
  wires:
  MATLAB Function5/1(y) -> Grad/1
  State/1 -> Sum4/1
  Position/1 -> MATLAB Function2/2(pos)
  MATLAB Function2/1(y) -> Sum4/2
  Policy_SS1/1(NormOut) -> MATLAB Function5/1(u1)
  StartValue/1 -> MATLAB Function5/2(u2)
  [GradConst] -> MATLAB Function5/3(const)
  Sum4/1 -> Policy_SS1/1(NormData)
  [GradConst] -> MATLAB Function2/1(u)

== system RealLifeTrainModel/ContractionMetricFilterSystem3/CalcK/IndidualGrad10 ==
  State : Inport
  Position : Inport  Port=2
  StartValue : Inport  Port=3
  MATLAB Function2 : MATLAB Function  TreatAsAtomicUnit=on
  MATLAB Function5 : MATLAB Function  TreatAsAtomicUnit=on
  Policy_SS1 : Subsystem
  Sum4 : Sum  Inputs=|++
  Grad : Outport
  wires:
  [GradConst] -> MATLAB Function5/3(const)
  Sum4/1 -> Policy_SS1/1(NormData)
  Policy_SS1/1(NormOut) -> MATLAB Function5/1(u1)
  [GradConst] -> MATLAB Function2/1(u)
  State/1 -> Sum4/1
  MATLAB Function2/1(y) -> Sum4/2
  Position/1 -> MATLAB Function2/2(pos)
  MATLAB Function5/1(y) -> Grad/1
  StartValue/1 -> MATLAB Function5/2(u2)

== system RealLifeTrainModel/ContractionMetricFilterSystem3/CalcK/IndidualGrad2 ==
  State : Inport
  Position : Inport  Port=2
  StartValue : Inport  Port=3
  MATLAB Function2 : MATLAB Function  TreatAsAtomicUnit=on
  MATLAB Function5 : MATLAB Function  TreatAsAtomicUnit=on
  Policy_SS1 : Subsystem
  Sum4 : Sum  Inputs=|++
  Grad : Outport
  wires:
  MATLAB Function5/1(y) -> Grad/1
  State/1 -> Sum4/1
  Position/1 -> MATLAB Function2/2(pos)
  MATLAB Function2/1(y) -> Sum4/2
  Policy_SS1/1(NormOut) -> MATLAB Function5/1(u1)
  StartValue/1 -> MATLAB Function5/2(u2)
  [GradConst] -> MATLAB Function5/3(const)
  Sum4/1 -> Policy_SS1/1(NormData)
  [GradConst] -> MATLAB Function2/1(u)

== system RealLifeTrainModel/ContractionMetricFilterSystem3/CalcK/IndidualGrad3 ==
  State : Inport
  Position : Inport  Port=2
  StartValue : Inport  Port=3
  MATLAB Function2 : MATLAB Function  TreatAsAtomicUnit=on
  MATLAB Function5 : MATLAB Function  TreatAsAtomicUnit=on
  Policy_SS1 : Subsystem
  Sum4 : Sum  Inputs=|++
  Grad : Outport
  wires:
  MATLAB Function5/1(y) -> Grad/1
  State/1 -> Sum4/1
  Position/1 -> MATLAB Function2/2(pos)
  MATLAB Function2/1(y) -> Sum4/2
  Policy_SS1/1(NormOut) -> MATLAB Function5/1(u1)
  StartValue/1 -> MATLAB Function5/2(u2)
  [GradConst] -> MATLAB Function5/3(const)
  Sum4/1 -> Policy_SS1/1(NormData)
  [GradConst] -> MATLAB Function2/1(u)

== system RealLifeTrainModel/ContractionMetricFilterSystem3/CalcK/IndidualGrad4 ==
  State : Inport
  Position : Inport  Port=2
  StartValue : Inport  Port=3
  MATLAB Function2 : MATLAB Function  TreatAsAtomicUnit=on
  MATLAB Function5 : MATLAB Function  TreatAsAtomicUnit=on
  Policy_SS1 : Subsystem
  Sum4 : Sum  Inputs=|++
  Grad : Outport
  wires:
  MATLAB Function5/1(y) -> Grad/1
  State/1 -> Sum4/1
  Position/1 -> MATLAB Function2/2(pos)
  MATLAB Function2/1(y) -> Sum4/2
  Policy_SS1/1(NormOut) -> MATLAB Function5/1(u1)
  StartValue/1 -> MATLAB Function5/2(u2)
  [GradConst] -> MATLAB Function5/3(const)
  Sum4/1 -> Policy_SS1/1(NormData)
  [GradConst] -> MATLAB Function2/1(u)

== system RealLifeTrainModel/ContractionMetricFilterSystem3/CalcK/IndidualGrad5 ==
  State : Inport
  Position : Inport  Port=2
  StartValue : Inport  Port=3
  MATLAB Function2 : MATLAB Function  TreatAsAtomicUnit=on
  MATLAB Function5 : MATLAB Function  TreatAsAtomicUnit=on
  Policy_SS1 : Subsystem
  Sum4 : Sum  Inputs=|++
  Grad : Outport
  wires:
  MATLAB Function5/1(y) -> Grad/1
  State/1 -> Sum4/1
  Position/1 -> MATLAB Function2/2(pos)
  MATLAB Function2/1(y) -> Sum4/2
  Policy_SS1/1(NormOut) -> MATLAB Function5/1(u1)
  StartValue/1 -> MATLAB Function5/2(u2)
  [GradConst] -> MATLAB Function5/3(const)
  Sum4/1 -> Policy_SS1/1(NormData)
  [GradConst] -> MATLAB Function2/1(u)

== system RealLifeTrainModel/ContractionMetricFilterSystem3/CalcK/IndidualGrad6 ==
  State : Inport
  Position : Inport  Port=2
  StartValue : Inport  Port=3
  MATLAB Function2 : MATLAB Function  TreatAsAtomicUnit=on
  MATLAB Function5 : MATLAB Function  TreatAsAtomicUnit=on
  Policy_SS1 : Subsystem
  Sum4 : Sum  Inputs=|++
  Grad : Outport
  wires:
  MATLAB Function5/1(y) -> Grad/1
  State/1 -> Sum4/1
  Position/1 -> MATLAB Function2/2(pos)
  MATLAB Function2/1(y) -> Sum4/2
  Policy_SS1/1(NormOut) -> MATLAB Function5/1(u1)
  StartValue/1 -> MATLAB Function5/2(u2)
  [GradConst] -> MATLAB Function5/3(const)
  Sum4/1 -> Policy_SS1/1(NormData)
  [GradConst] -> MATLAB Function2/1(u)

== system RealLifeTrainModel/ContractionMetricFilterSystem3/CalcK/IndidualGrad7 ==
  State : Inport
  Position : Inport  Port=2
  StartValue : Inport  Port=3
  MATLAB Function2 : MATLAB Function  TreatAsAtomicUnit=on
  MATLAB Function5 : MATLAB Function  TreatAsAtomicUnit=on
  Policy_SS1 : Subsystem
  Sum4 : Sum  Inputs=|++
  Grad : Outport
  wires:
  MATLAB Function5/1(y) -> Grad/1
  State/1 -> Sum4/1
  Position/1 -> MATLAB Function2/2(pos)
  MATLAB Function2/1(y) -> Sum4/2
  Policy_SS1/1(NormOut) -> MATLAB Function5/1(u1)
  StartValue/1 -> MATLAB Function5/2(u2)
  [GradConst] -> MATLAB Function5/3(const)
  Sum4/1 -> Policy_SS1/1(NormData)
  [GradConst] -> MATLAB Function2/1(u)

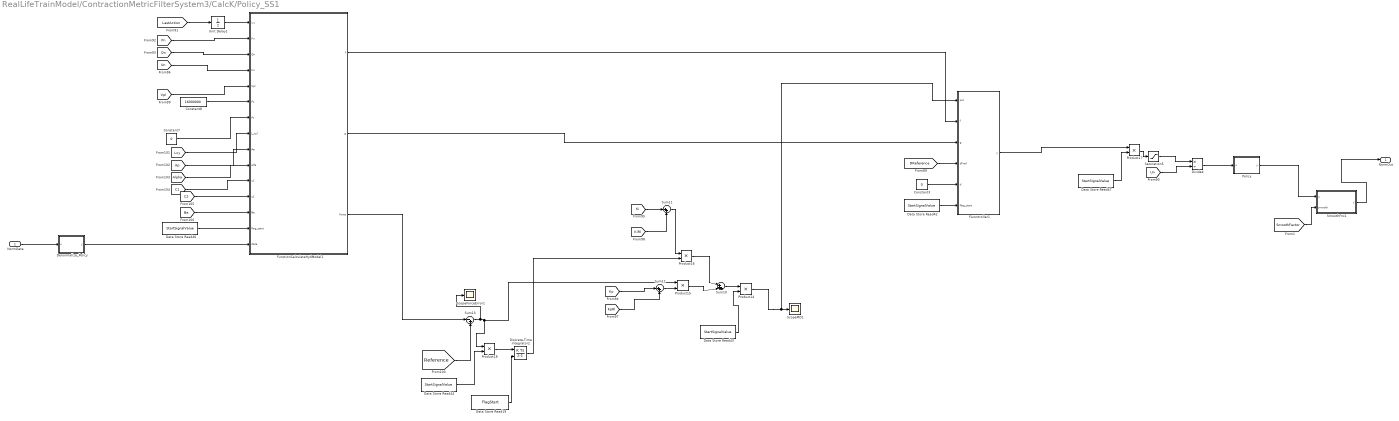
== system RealLifeTrainModel/ContractionMetricFilterSystem3/CalcK/Policy_SS1 ==
  NormData : Inport
  Constant3 : Constant  Value=0
  Constant7 : Constant  Value=0
  Constant8 : Constant  Value=16000000
  Data Store Read19 : DataStoreRead  DataStoreName=FlagStart  IndexOptions=Index vector (dialog)  Indices=1  OutputSizes=1
  Data Store Read{42..44,46..47} (5 alike) : DataStoreRead  DataStoreName=StartSignalValue  IndexOptions=Index vector (dialog)  Indices=1  OutputSizes=1
  Denormalize_Policy : MATLAB Function  TreatAsAtomicUnit=on
  Discrete-Time Integrator2 : DiscreteIntegrator  ExternalReset=either  SampleTime=-1  ICPrevOutput=DiscIntNeverNeededParam  ICPrevScaledInput=DiscIntNeverNeededParam
  Divide4 : Product  Inputs=*/
  FLcontroller1 : MATLAB Function  TreatAsAtomicUnit=on
  FunctionCalculateHydModel1 : MATLAB Function  TreatAsAtomicUnit=on
  Policy : MATLAB Function  TreatAsAtomicUnit=on
  Product{14..18} (5 alike) : Product
  Saturation5 : Saturate  UpperLimit=str2num(get_param('Teste_PID/Un','Value'))/str2num(get_param('Teste_PID/SaturationDivider','Value'))  LowerLimit=-str2num(get_param('Teste_PID/Un','Value'))/str2num(get_param('Teste_PID/SaturationDivider','Value'))
  ScopeForceError1 : Scope
  ScopePID1 : Scope
  SmoothFnc1 : MATLAB Function  TreatAsAtomicUnit=on
  Sum10 : Sum  Inputs=|+++
  Sum11 : Sum  Inputs=|++
  Sum12 : Sum  Inputs=|++
  Sum13 : Sum  Inputs=|-+
  Unit Delay1 : UnitDelay  SampleTime=-1  HasFrameUpgradeWarning=on
  NormOut : Outport
  wires:
  FunctionCalculateHydModel1/3(force) -> Sum13/1
  [Vpl] -> FunctionCalculateHydModel1/5(Vpl)
  Sum13/1 -> ScopeForceError1/1, Product15/1, Product18/1
  [Alpha] -> FunctionCalculateHydModel1/10(alfa)
  [C2] -> FunctionCalculateHydModel1/12(c2)
  Data Store Read42/1 -> FLcontroller1/6(flag_start)
  [Be] -> FunctionCalculateHydModel1/13(Be)
  [Lcy] -> FunctionCalculateHydModel1/8(L_cyl)
  Data Store Read43/1 -> Product14/2
  [Ap] -> FunctionCalculateHydModel1/9(Aa)
  Product15/1 -> Sum10/2
  Data Store Read44/1 -> Product18/2
  Product18/1 -> Discrete-Time Integrator2/1
  [KpRl] -> Sum12/2
  [Reference] -> Sum13/2
  Constant8/1 -> FunctionCalculateHydModel1/6(Ps)
  Product14/1 -> FLcontroller1/1(pid), ScopePID1/1
  Sum11/1 -> Product16/1
  Sum12/1 -> Product15/2
  Saturation5/1 -> Divide4/1
  [Un] -> Divide4/2
  FLcontroller1/1(y) -> Product17/1
  Denormalize_Policy/1(y) -> FunctionCalculateHydModel1/15(data)
  Sum10/1 -> Product14/1
  [C1] -> FunctionCalculateHydModel1/11(c1)
  Discrete-Time Integrator2/1 -> Product16/2
  [Pn] -> FunctionCalculateHydModel1/2(Pn)
  [LastAction] -> Unit Delay1/1
  [Kp] -> Sum12/1
  [Ki] -> Sum11/1
  Constant7/1 -> FunctionCalculateHydModel1/7(Pt)
  Divide4/1 -> Policy/1(u)
  [Qn] -> FunctionCalculateHydModel1/3(Qn)
  Constant3/1 -> FLcontroller1/5(d)
  [KiRl] -> Sum11/2
  Data Store Read47/1 -> Product17/2
  Product16/1 -> Sum10/1
  FunctionCalculateHydModel1/2(g) -> FLcontroller1/3(g)
  Product17/1 -> Saturation5/1
  [DReference] -> FLcontroller1/4(dFref)
  FunctionCalculateHydModel1/1(f) -> FLcontroller1/2(f)
  [Un] -> FunctionCalculateHydModel1/4(Un)
  Data Store Read46/1 -> FunctionCalculateHydModel1/14(flag_start)
  NormData/1 -> Denormalize_Policy/1(u)
  Unit Delay1/1 -> FunctionCalculateHydModel1/1(ixv)
  SmoothFnc1/1(y) -> NormOut/1
  Policy/1(y) -> SmoothFnc1/1(u)
  [SmoothFactor] -> SmoothFnc1/2(smooth)
  Data Store Read19/1 -> Discrete-Time Integrator2/2

== system RealLifeTrainModel/ContractionMetricFilterSystem3/Calc_A_B/Calc_A_Grad ==
  State : Inport
  Curent : Inport  Port=2
  Constant : Constant
  Constant1 : Constant  Value=2
  Constant2 : Constant  Value=3
  Constant3 : Constant  Value=4
  Constant4 : Constant  Value=5
  Constant5 : Constant  Value=6
  Constant6 : Constant  Value=7
  Constant7 : Constant  Value=8
  Constant8 : Constant  Value=9
  Data Type Conversion1 : DataTypeConversion  OutDataTypeStr=single  SaturateOnIntegerOverflow=off  RndMeth=Floor
  Data Type Conversion2 : DataTypeConversion  OutDataTypeStr=single  SaturateOnIntegerOverflow=off  RndMeth=Floor
  DynamicsConvert : MATLAB Function  TreatAsAtomicUnit=on
  IndidualGrad1 : Subsystem
  IndidualGrad10 : Subsystem
  IndidualGrad2 : Subsystem
  IndidualGrad3 : Subsystem
  IndidualGrad4 : Subsystem
  IndidualGrad5 : Subsystem
  IndidualGrad6 : Subsystem
  IndidualGrad7 : Subsystem
  IndidualGrad8 : Subsystem
  Mux : Mux  Inputs=8
  Mux1 : Mux  Inputs=2
  Reshape : Reshape  OutputDimensionality=Customize  OutputDimensions=[8,8]
  Reshape1 : Reshape  OutputDimensionality=Customize  OutputDimensions=[8,1]
  Scope : Scope
  Scope1 : Scope
  SubsystemModel : Subsystem
  A : Outport
  B : Outport  Port=2
  ModelPredict : Outport  Port=3
  wires:
  Mux/1 -> Reshape/1
  IndidualGrad10/1(Grad) -> Scope/1, Mux/1
  State/1 -> Mux1/1
  Curent/1 -> Mux1/2
  Data Type Conversion2/1 -> SubsystemModel/1(u), DynamicsConvert/1(x)
  Mux1/1 -> Data Type Conversion2/1, IndidualGrad8/1(State), IndidualGrad7/1(State), IndidualGrad6/1(State), IndidualGrad5/1(State), IndidualGrad4/1(State), IndidualGrad3/1(State), IndidualGrad2/1(State), IndidualGrad1/1(State), IndidualGrad10/1(State)
  Constant/1 -> IndidualGrad10/2(Position)
  Constant1/1 -> IndidualGrad1/2(Position)
  IndidualGrad1/1(Grad) -> Mux/2
  IndidualGrad7/1(Grad) -> Mux/8
  Constant7/1 -> IndidualGrad7/2(Position)
  Constant6/1 -> IndidualGrad6/2(Position)
  IndidualGrad6/1(Grad) -> Mux/7
  IndidualGrad5/1(Grad) -> Mux/6
  Constant5/1 -> IndidualGrad5/2(Position)
  IndidualGrad4/1(Grad) -> Mux/5
  Constant4/1 -> IndidualGrad4/2(Position)
  IndidualGrad2/1(Grad) -> Mux/3
  IndidualGrad3/1(Grad) -> Mux/4
  Constant2/1 -> IndidualGrad2/2(Position)
  Constant3/1 -> IndidualGrad3/2(Position)
  Constant8/1 -> IndidualGrad8/2(Position)
  Reshape/1 -> A/1
  Reshape1/1 -> B/1
  DynamicsConvert/1(dstate) -> Data Type Conversion1/1
  SubsystemModel/1(y) -> DynamicsConvert/2(y_model)
  [DiscreteContinousMode] -> DynamicsConvert/3(useDerivative)
  Data Type Conversion1/1 -> Scope1/1, ModelPredict/1, IndidualGrad8/3(StartValue), IndidualGrad7/3(StartValue), IndidualGrad6/3(StartValue), IndidualGrad5/3(StartValue), IndidualGrad4/3(StartValue), IndidualGrad3/3(StartValue), IndidualGrad2/3(StartValue), IndidualGrad1/3(StartValue), IndidualGrad10/3(StartValue)
  IndidualGrad8/1(Grad) -> Reshape1/1

== system RealLifeTrainModel/ContractionMetricFilterSystem3/Mdot_subsystem/IndidualGrad1 ==
  State : Inport
  Position : Inport  Port=2
  StartValue : Inport  Port=3
  ConvertMatrix : MATLAB Function  TreatAsAtomicUnit=on
  Data Type Conversion1 : DataTypeConversion  OutDataTypeStr=single  SaturateOnIntegerOverflow=off  RndMeth=Floor
  Data Type Conversion2 : DataTypeConversion  OutDataTypeStr=single  SaturateOnIntegerOverflow=off  RndMeth=Floor
  MATLAB Function2 : MATLAB Function  TreatAsAtomicUnit=on
  MATLAB Function5 : MATLAB Function  TreatAsAtomicUnit=on
  PredictMetric : deeplib/Predict  Network=Network from MAT-file  NetworkFunction=squeezenet  NetworkFilePath=C:\Users\ic2d\Documents\GitHub\dSpace_Controllers_legged\metric.mat  MiniBatchSize=128  InputDataFormats={'input', 'BC';}  Predictions=on  Activations={}  ForceInterpretedSim=off  EnableDLNetwork=on  LastKnownNetworkFilePath='C:\Users\ic2d\Documents\GitHub\dSpace_Controllers_legged\metric.mat'  LastKnownNetworkTimeStamp=739864.429490740760229527950286865234375
  Sum4 : Sum  Inputs=|++
  Grad : Outport
  wires:
  PredictMetric/1 -> Data Type Conversion1/1
  MATLAB Function2/1(y) -> Sum4/2
  [GradConst] -> MATLAB Function5/3(const)
  Data Type Conversion2/1 -> PredictMetric/1
  [GradConst] -> MATLAB Function2/1(u)
  Position/1 -> MATLAB Function2/2(pos)
  Data Type Conversion1/1 -> ConvertMatrix/1(M_flat)
  State/1 -> Sum4/1
  StartValue/1 -> MATLAB Function5/2(u2)
  Sum4/1 -> Data Type Conversion2/1
  MATLAB Function5/1(y) -> Grad/1
  ConvertMatrix/1(M) -> MATLAB Function5/1(u1)

== system RealLifeTrainModel/ContractionMetricFilterSystem3/Mdot_subsystem/IndidualGrad10 ==
  State : Inport
  Position : Inport  Port=2
  StartValue : Inport  Port=3
  ConvertMatrix : MATLAB Function  TreatAsAtomicUnit=on
  Data Type Conversion1 : DataTypeConversion  OutDataTypeStr=single  SaturateOnIntegerOverflow=off  RndMeth=Floor
  Data Type Conversion2 : DataTypeConversion  OutDataTypeStr=single  SaturateOnIntegerOverflow=off  RndMeth=Floor
  MATLAB Function2 : MATLAB Function  TreatAsAtomicUnit=on
  MATLAB Function5 : MATLAB Function  TreatAsAtomicUnit=on
  PredictMetric : deeplib/Predict  Network=Network from MAT-file  NetworkFunction=squeezenet  NetworkFilePath=C:\Users\ic2d\Documents\GitHub\dSpace_Controllers_legged\metric.mat  MiniBatchSize=128  InputDataFormats={'input', 'BC';}  Predictions=on  Activations={}  ForceInterpretedSim=off  EnableDLNetwork=on  LastKnownNetworkFilePath='C:\Users\ic2d\Documents\GitHub\dSpace_Controllers_legged\metric.mat'  LastKnownNetworkTimeStamp=739864.429490740760229527950286865234375
  Sum4 : Sum  Inputs=|++
  Grad : Outport
  wires:
  [GradConst] -> MATLAB Function5/3(const)
  [GradConst] -> MATLAB Function2/1(u)
  State/1 -> Sum4/1
  MATLAB Function2/1(y) -> Sum4/2
  Position/1 -> MATLAB Function2/2(pos)
  MATLAB Function5/1(y) -> Grad/1
  StartValue/1 -> MATLAB Function5/2(u2)
  PredictMetric/1 -> Data Type Conversion1/1
  Data Type Conversion2/1 -> PredictMetric/1
  Sum4/1 -> Data Type Conversion2/1
  Data Type Conversion1/1 -> ConvertMatrix/1(M_flat)
  ConvertMatrix/1(M) -> MATLAB Function5/1(u1)
